simulink model "Mini_project_sim_2020"  (R2020b)
settings: Solver=ode113  StartTime=0.0  StopTime=10  FixedStep=0.001  RelTol=0.0001
values from neighbouring files (symbols this model uses):
  A = [0 1 0 0; 0.0290 0 7.0062 0; 0 0 0 1; -3.1991 0 0.1088 0]    [BallBeam3.m]
  B = [0; -4.332; 0; 47.7514]    [BallBeam3.m]
  C = [1 0 0 0;  0 0 1 0]    [BallBeam3.m]
  g = 9.81    [BallBeam3.m]
  ica = 0.1    [BallBeam3.m]
  icx = L/2    (= 0.21275)    [BallBeam3.m]
  J = 0.02    [BallBeam3.m]
  K = lqr(A,B,Q,R)    [BallBeam3.m]
  L = 0.4255    [BallBeam3.m]
  Lo = place(A', C', full_state_poles .* 10)'    [BallBeam3.m]
  m = 0.064    [BallBeam3.m]
  r = 0.0127    [BallBeam3.m]
  R = 1    [BallBeam3.m]
  step_input_value = 0.1    [BallBeam3.m]
undefined symbols (not defined in the file or in its folder): FSFB, K_Bar, Kd, Ki, Kp, observer_L, tau
libraries: simulink x2, dspsrcs4 x2
settings Model: Creator=jackg  LastModifiedBy=Andreas Wiedholz
settings SolverCC: MaxConsecutiveMinStep=500
settings DebuggingCC: SFMachineParentedDataDiag=error  UnderSpecifiedDimensionMsg=warning

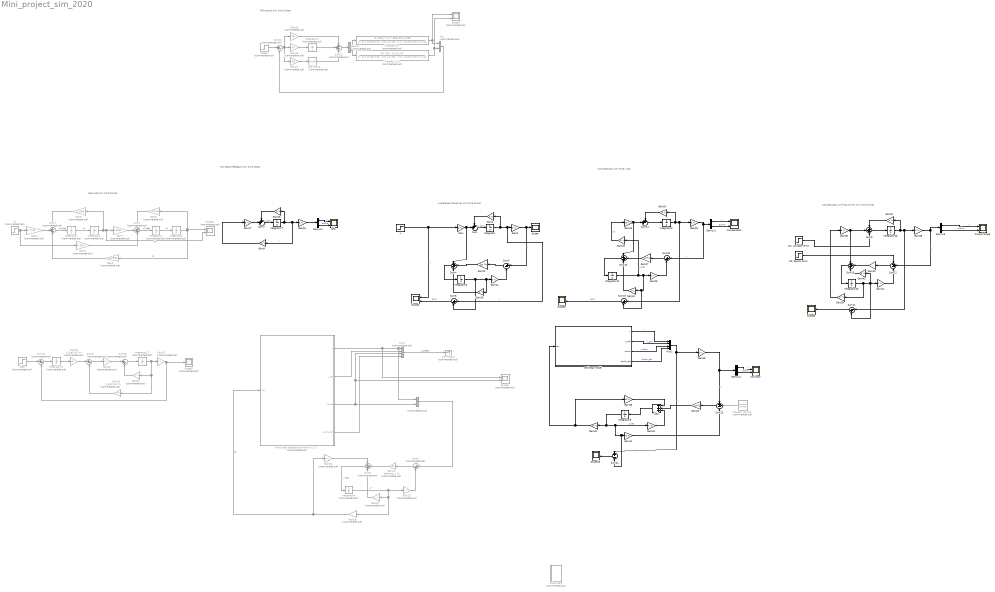
== system Mini_project_sim_2020 ==
  note: open loop sim time 10 sec
  note: Full State Feedback sim time 10sec
  note: Luenberger Observer sim time 10 sec
  note: Compensator sim time 1 sec
  note: Compensator with S/A errors sim time 10 sec
  note: PID control sim time 10sec
  AZ- Actuator error : Step  Time=0  After=[0; 0; 0.01; 0]  SampleTime=0
  Add : Sum  Inputs=+++
  Demux : Demux  Commented=on  Outputs=2
  Demux{1..4} (4 alike) : Demux  Outputs=2
  Derivative : Derivative  Commented=on
  Gain{,17,23,35..36} (5 alike) : Gain  Gain=B  Multiplication=Matrix(K*u)
  Gain{1,10,15,24,34,37,42..43} (8 alike) : Gain  Gain=A  Multiplication=Matrix(K*u)
  Gain{2,11,16,25,28,38,41,44,49} (9 alike) : Gain  Gain=C  Multiplication=Matrix(K*u)
  Gain{12,22,27,40} (4 alike) : Gain  Gain=Lo  Multiplication=Matrix(K*u)
  Gain13 : Gain  Commented=on  Gain=C  Multiplication=Matrix(K*u)
  Gain14 : Gain  Commented=on  Gain=observer_L  Multiplication=Matrix(K*u)
  Gain18 : Gain  Commented=on  Gain=B  Multiplication=Matrix(K*u)
  Gain19 : Gain  Commented=on  Gain=-FSFB  Multiplication=Matrix(K*u)
  Gain20 : Gain  Commented=on  Gain=A  Multiplication=Matrix(K*u)
  Gain{9,26,39,48} (4 alike) : Gain  Gain=-K  Multiplication=Matrix(K*u)
  Gain29 : Gain  Commented=on  Gain=K_Bar(5:6)  Multiplication=Matrix(K*u)
  Gain3 : Gain  Commented=on  Gain=3.1991
  Gain30 : Gain  Commented=on  Gain=B  Multiplication=Matrix(K*u)
  Gain31 : Gain  Commented=on  Gain=C  Multiplication=Matrix(K*u)
  Gain32 : Gain  Commented=on  Gain=A  Multiplication=Matrix(K*u)
  Gain33 : Gain  Commented=on  Gain=K_Bar(1:4)  Multiplication=Matrix(K*u)
  Gain4 : Gain  Commented=on  Gain=47.7514
  Gain45 : Gain  Commented=on  Gain=Kp
  Gain46 : Gain  Commented=on  Gain=Ki
  Gain47 : Gain  Commented=on  Gain=Kd
  Gain5 : Gain  Commented=on  Gain=0.1088
  Gain6 : Gain  Commented=on  Gain=4.332
  Gain7 : Gain  Commented=on  Gain=7.0062
  Gain8 : Gain  Commented=on  Gain=0.0290
  Integrator : Integrator
  Integrator{1..4,11..12,17} (7 alike) : Integrator  Commented=on
  Integrator10 : Integrator  InitialCondition=[0.1;0;0;0]
  Integrator15 : Integrator  InitialCondition=[0.1,0,0,0]
  Integrator16 : Integrator  InitialCondition=[icx;0;ica;0]
  Integrator5 : Integrator
  Integrator6 : Integrator  Commented=on  InitialCondition=[0;0;0;0]
  Integrator7 : Integrator  InitialCondition=[icx; 0;ica;0]
  Integrator8 : Integrator  InitialCondition=[0.1;0;0;0]
  Integrator9 : Integrator  InitialCondition=[icx;0;ica;0]
  Mux : Mux  Commented=on  Inputs=2
  Mux1 : Mux  Commented=on
  Mux2 : Mux
  "Non-Linear equations of motion 1 & 2 " : Subsystem  Commented=on
  Output Scope : Scope  NumInputPorts=2
  Random Source : dspsrcs4/Random Source  Commented=on  SrcType=Uniform  NormMethod=Ziggurat  CltLength=12  MinVal=[-0.01; -0.01]  MaxVal=[0.01; 0.01]  MeanVal=0  VarVal=1  RepMode=Not repeatable  rawSeed=1  IsInherit=off  SampMode=Discrete  SampTime=1  SampFrame=1  DataType=Double  OutComplex=Real  OutputFrames=off
  Scope{,6,8,10} (4 alike) : Scope
  Scope1 : Scope  Commented=on  NumInputPorts=2
  Scope2 : Scope  NumInputPorts=2
  Scope3 : Scope  Commented=on
  Scope5 : Scope  Commented=on  NumInputPorts=2
  Scope9 : Scope  Commented=on  NumInputPorts=4
  Step : Step  Commented=on  After=R  SampleTime=0
  Step3 : Step  Commented=on  SampleTime=0
  Subsystem : Subsystem  Commented=on
  Sum : Sum  Inputs=++|
  Sum1 : Sum  Commented=on  Inputs=++-
  Sum10 : Sum  Inputs=+++
  Sum11 : Sum  Inputs=|-+
  Sum12 : Sum  Inputs=-+-
  Sum13 : Sum  Inputs=++-
  Sum14 : Sum  Inputs=++|
  Sum15 : Sum  Inputs=+++
  Sum{3,16..17,21} (4 alike) : Sum  Commented=on  Inputs=|+-
  Sum18 : Sum  Commented=on  Inputs=|++
  Sum19 : Sum  Inputs=|+-
  Sum2 : Sum  Commented=on  Inputs=++-
  Sum20 : Sum  Inputs=|+-
  Sum22 : Sum  Commented=on  Inputs=+++
  Sum24 : Sum  Inputs=+-
  Sum4 : Sum  Inputs=+++
  Sum5 : Sum  Inputs=|+-  OutDataTypeStr=Inherit: Same as accumulator
  Sum6 : Sum  Inputs=|+-
  Sum7 : Sum  Inputs=++|
  Sum8 : Sum  Commented=on  Inputs=+++
  Sum9 : Sum  Inputs=++-
  Terminator : Terminator  Commented=on
  Transfer Fcn : TransferFcn  Commented=on  Numerator=[-4.332 7.69e-15 335]  Denominator=[1 -3.553e-15 -0.1378 1.332e-14 22.42]
  Transfer Fcn1 : TransferFcn  Commented=on  Numerator=[47.75 0 12.47]  Denominator=[1 -3.553e-15 -0.1378 1.332e-14 22.42]
  ZS- Sensor error : Step  Time=0  After=[-0.05 0]  SampleTime=0
  compensator : Scope  NumInputPorts=2
  fsfb : Scope  NumInputPorts=2
  nonlinear : Scope  NumInputPorts=2
  nonlinear model : Subsystem
  u : Step  After=step_input_value  SampleTime=0
  u1 : Step  Commented=on  SampleTime=0
  y : Mux  Commented=on  Inputs=2
  wires:
  Integrator/1 -> Sum6/1, Gain2/1, Gain1/1  "x"
  Sum/1 -> Integrator/1  "x_dot"
  Gain1/1 -> Sum/1
  Gain/1 -> Sum4/1, Sum/2
  Gain2/1 -> Sum5/1, Scope/1  "y"
  Integrator1/1 -> Integrator2/1  "x4"
  Integrator2/1 -> Scope1/2, Gain7/1, Gain5/1  "x3"
  Integrator3/1 -> Integrator4/1  "x2"
  Sum1/1 -> Integrator1/1  "x4_dot"
  Integrator4/1 -> Scope1/1, Gain8/1, Gain3/1  "x1"
  Gain3/1 -> Sum1/3
  Gain4/1 -> Sum1/2
  u1/1 -> Gain6/1, Gain4/1
  Gain5/1 -> Sum1/1
  Sum2/1 -> Integrator3/1  "x2_dot"
  Gain6/1 -> Sum2/3
  Gain7/1 -> Sum2/2
  Gain8/1 -> Sum2/1
  u/1 -> Gain/1, Scope2/1  "u"
  Integrator5/1 -> Sum6/2, Gain10/1, Gain11/1
  Gain11/1 -> Sum5/2
  Sum5/1 -> Gain12/1
  Sum4/1 -> Integrator5/1
  Sum6/1 -> Scope2/2  "error"
  Gain10/1 -> Sum4/3
  Gain12/1 -> Sum4/2
  Integrator7/1 -> Gain9/1, Gain16/1, Gain15/1  "x"
  Sum7/1 -> Integrator7/1  "x_dot"
  Gain15/1 -> Sum7/1
  Gain17/1 -> Sum7/2
  Step/1 -> Sum16/1
  Sum16/1 -> Integrator11/1
  Integrator11/1 -> Gain29/1
  Gain29/1 -> Sum17/1
  Sum17/1 -> Gain30/1
  Gain30/1 -> Sum18/1
  Sum18/1 -> Integrator12/1
  Integrator12/1 -> Gain33/1, Gain32/1, Gain31/1
  Gain32/1 -> Sum18/2
  Gain31/1 -> Scope3/1, Sum16/2
  Gain33/1 -> Sum17/2
  Gain23/1 -> Sum15/1, Sum14/2
  Gain24/1 -> Sum14/1
  Sum14/1 -> Integrator9/1
  Integrator9/1 -> Gain24/1, Sum19/1, Gain25/1
  Gain25/1 -> Demux1/1, Sum20/1  "y"
  Gain27/1 -> Sum15/2
  Sum20/1 -> Gain27/1
  Gain28/1 -> Sum20/2
  Integrator10/1 -> Gain34/1, Sum19/2, Gain28/1, Gain26/1  "x_hat"
  Sum15/1 -> Integrator10/1
  Gain34/1 -> Sum15/3
  Sum19/1 -> Scope8/1  "error"
  Sum11/1 -> Scope6/1
  Gain42/1 -> Sum10/3
  Sum10/1 -> Integrator15/1
  Integrator15/1 -> Sum11/2, Gain42/1, Gain41/1, Gain39/1
  Sum12/1 -> Gain40/1
  Gain40/1 -> Sum10/2
  Gain38/1 -> Sum12/2, Demux3/1  "y"
  Integrator16/1 -> Gain38/1, Sum11/1, Gain37/1
  Sum9/1 -> Integrator16/1
  Gain37/1 -> Sum9/1
  Gain36/1 -> Sum9/2, Sum10/1
  Gain39/1 -> Gain36/1
  AZ- Actuator error/1 -> Sum9/3
  Gain41/1 -> Sum12/3
  ZS- Sensor error/1 -> Sum12/1
  Demux/2 -> Transfer Fcn1/1
  Demux/1 -> Transfer Fcn/1
  Transfer Fcn/1 -> Scope5/1, Mux/1
  Transfer Fcn1/1 -> Scope5/2, Mux/2
  Mux/1 -> Sum21/2
  Step3/1 -> Sum21/1
  Sum22/1 -> Demux/1
  Sum21/1 -> Gain45/1, Gain47/1, Gain46/1
  Gain47/1 -> Derivative/1
  Derivative/1 -> Sum22/3
  Integrator17/1 -> Sum22/2
  Gain45/1 -> Sum22/1
  Gain46/1 -> Integrator17/1
  Demux1/2 -> compensator/2  "alpha"
  Gain16/1 -> Demux2/1  "y"
  Demux2/1 -> fsfb/1  "x"
  Demux2/2 -> fsfb/2  "alpha"
  Demux1/1 -> compensator/1  "x"
  Gain9/1 -> Gain17/1
  Gain26/1 -> Gain23/1  "Lin"
  Demux3/1 -> Output Scope/1  "x"
  Demux3/2 -> Output Scope/2  "alpha"
  "Non-Linear equations of motion 1 & 2 "/1(x) -> Scope9/2, y/1, Mux1/1
  "Non-Linear equations of motion 1 & 2 "/2(x_dot) -> Mux1/2
  "Non-Linear equations of motion 1 & 2 "/3(alpha) -> y/2, Mux1/3, Scope9/3
  "Non-Linear equations of motion 1 & 2 "/4(alpha_dot) -> Mux1/4
  Mux1/1 -> Terminator/1  "x_vector"
  Gain13/1 -> Sum3/2
  Sum3/1 -> Gain14/1
  y/1 -> Sum3/1
  Gain14/1 -> Sum8/2
  Gain18/1 -> Sum8/1
  Gain19/1 -> Gain18/1, "Non-Linear equations of motion 1 & 2 "/1(Tau)  "NL"
  Integrator6/1 -> Gain13/1, Gain20/1, Gain19/1  "x^"
  Sum8/1 -> Integrator6/1  "x^dot"
  Gain20/1 -> Sum8/3
  Gain48/1 -> Gain35/1, nonlinear model/1(tau)
  Sum13/1 -> Gain22/1
  Integrator8/1 -> Gain43/1, Sum24/2, Gain44/1, Gain48/1  "x_hat"
  Gain44/1 -> Sum13/3
  nonlinear model/3(alpha) -> Mux2/3  "alpha"
  nonlinear model/4(alpha_dot) -> Mux2/4  "alpha_dot"
  Sum24/1 -> Scope10/1
  nonlinear model/2(x_dot) -> Mux2/2  "x_dot"
  nonlinear model/1(x) -> Mux2/1  "x"
  Mux2/1 -> Gain49/1, Sum24/1  "x"
  Gain35/1 -> Add/1
  Gain22/1 -> Add/2
  Gain43/1 -> Add/3
  Add/1 -> Integrator8/1
  Gain49/1 -> Sum13/1, Demux4/1  "y"
  Demux4/1 -> nonlinear/1  "x"
  Demux4/2 -> nonlinear/2  "alpha"
  Random Source/1 -> Sum13/2

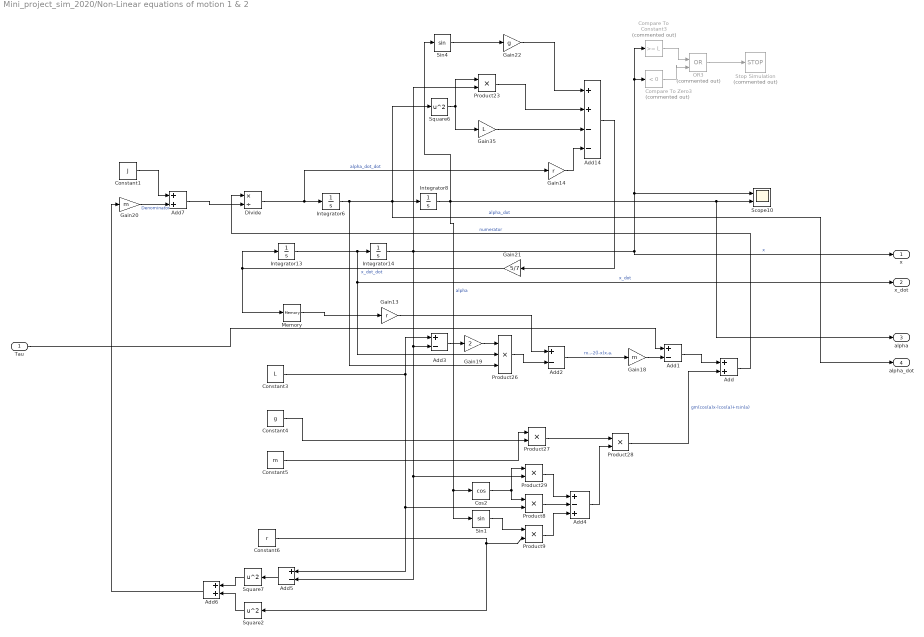
== system Mini_project_sim_2020/Non-Linear equations of motion 1 & 2  ==
  Tau : Inport
  Add : Sum
  Add{1..3,5} (4 alike) : Sum  Inputs=+-
  Add14 : Sum  Inputs=++--
  Add4 : Sum  Inputs=+-+
  Add6 : Sum
  Add7 : Sum
  Compare To Constant3 : simulink/Logic and Bit Operations/Compare To Constant  Commented=on  relop=>=  const=L  OutDataTypeStr=boolean
  Compare To Zero3 : simulink/Logic and Bit Operations/Compare To Zero  Commented=on  relop=<  OutDataTypeStr=boolean
  Constant1 : Constant  Value=J
  Constant3 : Constant  Value=L
  Constant4 : Constant  Value=g
  Constant5 : Constant  Value=m
  Constant6 : Constant  Value=r
  Cos2 : Trigonometry  Operator=cos
  Divide : Product  Inputs=*/
  Gain13 : Gain  Gain=r
  Gain14 : Gain  Gain=r
  Gain18 : Gain  Gain=m
  Gain19 : Gain  Gain=2
  Gain20 : Gain  Gain=m
  Gain21 : Gain  Gain=5/7
  Gain22 : Gain  Gain=g
  Gain35 : Gain  Gain=L
  Integrator13 : Integrator
  Integrator14 : Integrator  InitialCondition=L/2
  Integrator6 : Integrator
  Integrator8 : Integrator  InitialCondition=0.1
  Memory : Memory
  OR3 : Logic  Commented=on  Operator=OR  IconShape=distinctive  AllPortsSameDT=off  OutDataTypeStr=boolean
  Product{8..9,23,27..29} (6 alike) : Product
  Product26 : Product  Inputs=3
  Scope10 : Scope  NumInputPorts=2
  Sin1 : Trigonometry
  Sin4 : Trigonometry
  Square2 : Math  Operator=square  SaturateOnIntegerOverflow=on
  Square6 : Math  Operator=square  SaturateOnIntegerOverflow=on
  Square7 : Math  Operator=square  SaturateOnIntegerOverflow=on
  Stop Simulation : Stop  Commented=on
  x : Outport
  x_dot : Outport  Port=2
  alpha : Outport  Port=3
  alpha_dot : Outport  Port=4
  wires:
  Square7/1 -> Add6/1
  Integrator6/1 -> Product26/3, alpha_dot/1, Square6/1, Integrator8/1  "alpha_dot"
  Add7/1 -> Divide/2
  Divide/1 -> Gain14/1, Integrator6/1  "alpha_dot_dot"
  Sin4/1 -> Gain22/1
  Integrator8/1 -> Sin1/1, Cos2/1, alpha/1, Scope10/2, Sin4/1  "alpha"
  Add/1 -> Divide/1  "numerator"
  Gain35/1 -> Add14/3
  Gain14/1 -> Add14/4
  Compare To Constant3/1 -> OR3/1
  Square2/1 -> Add6/2
  Integrator14/1 -> Compare To Zero3/1, Compare To Constant3/1, Scope10/1, x/1, Product23/2, Add5/2, Product29/2, Add3/2  "x"
  Constant4/1 -> Product27/2
  OR3/1 -> Stop Simulation/1
  Constant6/1 -> Square2/1, Product9/2
  Gain19/1 -> Product26/1
  Integrator13/1 -> Integrator14/1, x_dot/1, Product26/2  "x_dot"
  Gain13/1 -> Add2/1
  Add1/1 -> Add/1
  Product9/1 -> Add4/3
  Constant5/1 -> Product27/1
  Gain20/1 -> Add7/2  "Denominator"
  Gain21/1 -> Memory/1, Integrator13/1  "x_dot_dot"
  Constant1/1 -> Add7/1
  Constant3/1 -> Add3/1, Add5/1, Product8/2
  Add5/1 -> Square7/1
  Product29/1 -> Add4/1
  Add6/1 -> Gain20/1
  Cos2/1 -> Product29/1, Product8/1
  Gain18/1 -> Add1/2
  Compare To Zero3/1 -> OR3/2
  Product8/1 -> Add4/2
  Add14/1 -> Gain21/1
  Add4/1 -> Product28/2
  Square6/1 -> Gain35/1, Product23/1
  Product26/1 -> Add2/2
  Sin1/1 -> Product9/1
  Add3/1 -> Gain19/1
  Product23/1 -> Add14/2
  Product27/1 -> Product28/1
  Gain22/1 -> Add14/1
  Add2/1 -> Gain18/1  "rx..-2(l-x)x.a."
  Product28/1 -> Add/2  "gm(cos(a)x-lcos(a)+rsin(a)"
  Memory/1 -> Gain13/1
  Tau/1 -> Add1/1

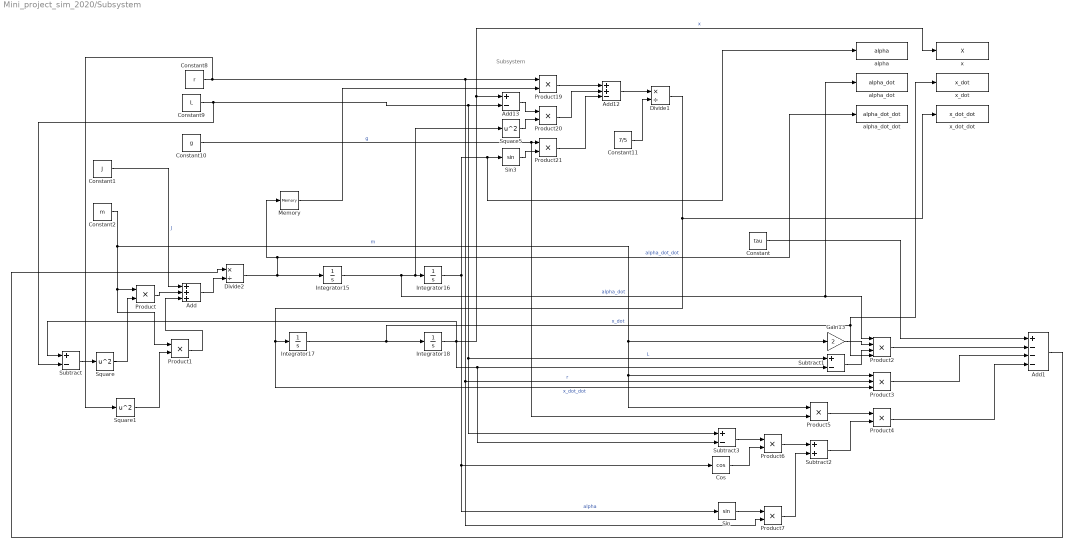
== system Mini_project_sim_2020/Subsystem ==
  note: Subsystem
  Add : Sum  Inputs=+++
  Add1 : Sum  Inputs=+---
  Add12 : Sum  Inputs=++-
  Add13 : Sum  Inputs=+-
  Constant : Constant  Value=tau
  Constant1 : Constant  Value=J
  Constant10 : Constant  Value=g
  Constant11 : Constant  Value=7/5
  Constant2 : Constant  Value=m
  Constant8 : Constant  Value=r
  Constant9 : Constant  Value=L
  Cos : Trigonometry  Operator=cos
  Divide1 : Product  Inputs=*/
  Divide2 : Product  Inputs=*/
  Gain13 : Gain  Gain=2
  Integrator{15..18} (4 alike) : Integrator
  Memory : Memory
  Product{,1,4..7,19..21} (9 alike) : Product
  Product2 : Product  Inputs=4
  Product3 : Product  Inputs=3
  Sin : Trigonometry
  Sin3 : Trigonometry
  Square : Math  Operator=square  SaturateOnIntegerOverflow=on
  Square1 : Math  Operator=square  SaturateOnIntegerOverflow=on
  Square5 : Math  Operator=square  SaturateOnIntegerOverflow=on
  Subtract : Sum  Inputs=+-
  Subtract1 : Sum  Inputs=+-
  Subtract2 : Sum
  Subtract3 : Sum  Inputs=+-
  alpha : ToWorkspace  VariableName=alpha  SaveFormat=Timeseries  SampleTime=-1
  alpha_dot : ToWorkspace  VariableName=alpha_dot  SaveFormat=Timeseries  SampleTime=-1
  alpha_dot_dot : ToWorkspace  VariableName=alpha_dot_dot  SaveFormat=Timeseries  SampleTime=-1
  x : ToWorkspace  VariableName=X  SaveFormat=Timeseries  SampleTime=-1
  x_dot : ToWorkspace  VariableName=x_dot  SaveFormat=Timeseries  SampleTime=-1
  x_dot_dot : ToWorkspace  VariableName=x_dot_dot  SaveFormat=Timeseries  SampleTime=-1
  wires:
  Integrator15/1 -> alpha_dot/1, Product2/1, Square5/1, Integrator16/1  "alpha_dot"
  Divide2/1 -> Memory/1, alpha_dot_dot/1, Integrator15/1  "alpha_dot_dot"
  Constant8/1 -> Square1/1, Product7/2, Product3/2, Product19/1  "r"
  Subtract/1 -> Square/1
  Sin3/1 -> Product21/2
  Integrator18/1 -> Subtract3/2, Subtract1/2, Subtract/1, x/1, Add13/1  "x"
  Product2/1 -> Add1/2
  Constant1/1 -> Add/1  "J"
  Divide1/1 -> x_dot_dot/1, Product3/3, Integrator17/1  "x_dot_dot"
  Square1/1 -> Product1/2
  Add13/1 -> Product20/1
  Constant10/1 -> Product5/2, Product21/1  "g"
  Constant9/1 -> Subtract/2, Subtract3/1, Subtract1/1, Add13/2  "L"
  Constant/1 -> Add1/1
  Square/1 -> Product/2
  Gain13/1 -> Product2/2
  Product7/1 -> Subtract2/2
  Constant2/1 -> Product5/1, Product3/1, Gain13/1, Product1/1, Product/1  "m"
  Constant11/1 -> Divide1/2
  Product3/1 -> Add1/3
  Product/1 -> Add/2
  Integrator16/1 -> alpha/1, Sin3/1, Cos/1, Sin/1  "alpha"
  Integrator17/1 -> x_dot/1, Product2/4, Integrator18/1  "x_dot"
  Subtract3/1 -> Product6/1
  Product21/1 -> Add12/3
  Cos/1 -> Product6/2
  Product19/1 -> Add12/1
  Product6/1 -> Subtract2/1
  Sin/1 -> Product7/1
  Product1/1 -> Add/3
  Subtract2/1 -> Product4/2
  Add12/1 -> Divide1/1
  Product20/1 -> Add12/2
  Add/1 -> Divide2/2
  Product4/1 -> Add1/4
  Square5/1 -> Product20/2
  Product5/1 -> Product4/1
  Add1/1 -> Divide2/1
  Subtract1/1 -> Product2/3
  Memory/1 -> Product19/2

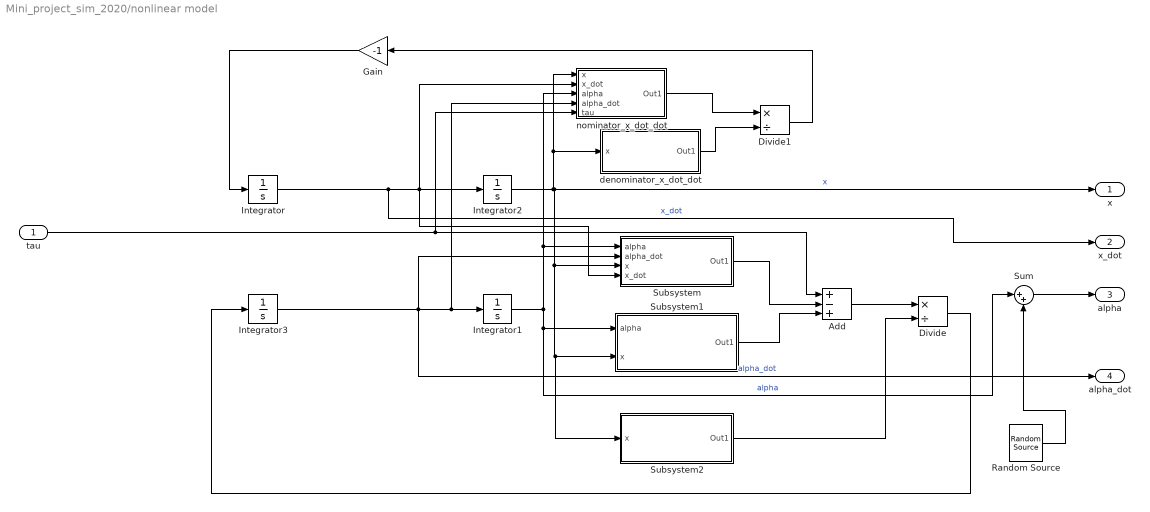
== system Mini_project_sim_2020/nonlinear model ==
  tau : Inport
  Add : Sum  Inputs=+-+
  Divide : Product  Inputs=*/
  Divide1 : Product  Inputs=*/
  Gain : Gain  Gain=-1
  Integrator : Integrator
  Integrator1 : Integrator  InitialCondition=0.1
  Integrator2 : Integrator  InitialCondition=L/2
  Integrator3 : Integrator
  Random Source : dspsrcs4/Random Source  SrcType=Uniform  NormMethod=Ziggurat  CltLength=12  MinVal=-0.01  MaxVal=0.02  MeanVal=0  VarVal=1  RepMode=Not repeatable  rawSeed=1  IsInherit=off  SampMode=Discrete  SampTime=1  SampFrame=1  DataType=Double  OutComplex=Real  OutputFrames=off
  Subsystem : Subsystem
      mask Display: disp('m(r(5gsin(alpha)...))')
  Subsystem1 : Subsystem
      mask Display: disp('gm(cos(alpha)...)')
  Subsystem2 : Subsystem
      mask Display: disp('denominator')
  Sum : Sum  Inputs=|++
  denominator_x_dot_dot : Subsystem
      mask Display: disp('denominator')
  nominator_x_dot_dot : Subsystem
      mask Display: disp('nominator')
  x : Outport
  x_dot : Outport  Port=2
  alpha : Outport  Port=3
  alpha_dot : Outport  Port=4
  wires:
  Integrator/1 -> x_dot/1, nominator_x_dot_dot/2(x_dot), Subsystem/4(x_dot), Integrator2/1  "x_dot"
  Integrator3/1 -> alpha_dot/1, nominator_x_dot_dot/4(alpha_dot), Integrator1/1, Subsystem/2(alpha_dot)  "alpha_dot"
  Integrator1/1 -> Sum/1, Subsystem1/1(alpha), nominator_x_dot_dot/3(alpha), Subsystem/1(alpha)  "alpha"
  Integrator2/1 -> x/1, Subsystem/3(x), Subsystem2/1(x), Subsystem1/2(x), denominator_x_dot_dot/1(x), nominator_x_dot_dot/1(x)  "x"
  tau/1 -> nominator_x_dot_dot/5(tau), Add/1
  Subsystem/1(Out1) -> Add/2
  Subsystem1/1(Out1) -> Add/3
  Add/1 -> Divide/1
  Subsystem2/1(Out1) -> Divide/2
  Divide/1 -> Integrator3/1
  nominator_x_dot_dot/1(Out1) -> Divide1/1
  denominator_x_dot_dot/1(Out1) -> Divide1/2
  Divide1/1 -> Gain/1
  Gain/1 -> Integrator/1
  Sum/1 -> alpha/1
  Random Source/1 -> Sum/2

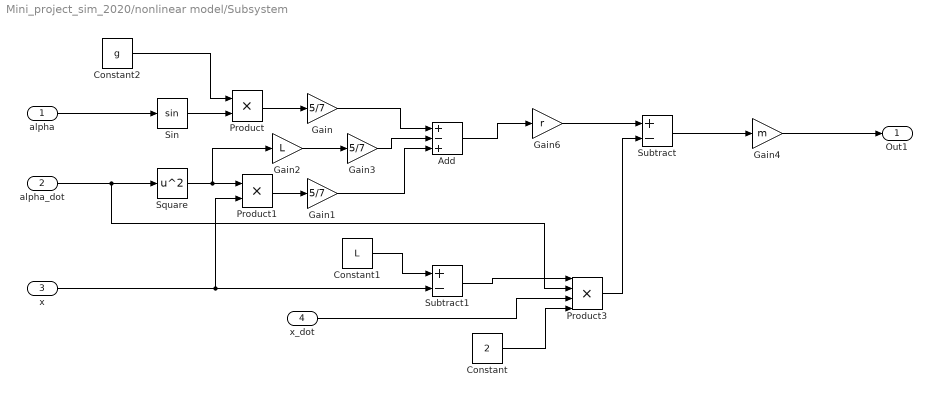
== system Mini_project_sim_2020/nonlinear model/Subsystem ==
  alpha : Inport
  alpha_dot : Inport  Port=2
  x : Inport  Port=3
  x_dot : Inport  Port=4
  Add : Sum  Inputs=+-+
  Constant : Constant  Value=2
  Constant1 : Constant  Value=L
  Constant2 : Constant  Value=g
  Gain : Gain  Gain=5/7
  Gain1 : Gain  Gain=5/7
  Gain2 : Gain  Gain=L
  Gain3 : Gain  Gain=5/7
  Gain4 : Gain  Gain=m
  Gain6 : Gain  Gain=r
  Product : Product
  Product1 : Product
  Product3 : Product  Inputs=4
  Sin : Trigonometry
  Square : Math  Operator=square  SaturateOnIntegerOverflow=on
  Subtract : Sum  Inputs=+-
  Subtract1 : Sum  Inputs=+-
  Out1 : Outport
  wires:
  alpha_dot/1 -> Product3/2, Square/1
  alpha/1 -> Sin/1
  Sin/1 -> Product/2
  Constant2/1 -> Product/1
  Product/1 -> Gain/1
  Square/1 -> Gain2/1, Product1/1
  x/1 -> Product1/2, Subtract1/2
  Product1/1 -> Gain1/1
  Gain2/1 -> Gain3/1
  Gain/1 -> Add/1
  Gain3/1 -> Add/2
  Gain1/1 -> Add/3
  Gain4/1 -> Out1/1
  Gain6/1 -> Subtract/1
  Constant1/1 -> Subtract1/1
  Subtract1/1 -> Product3/1
  x_dot/1 -> Product3/3
  Product3/1 -> Subtract/2
  Subtract/1 -> Gain4/1
  Add/1 -> Gain6/1
  Constant/1 -> Product3/4

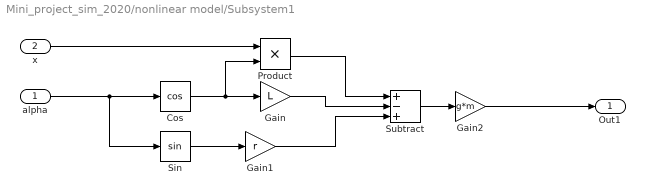
== system Mini_project_sim_2020/nonlinear model/Subsystem1 ==
  alpha : Inport
  x : Inport  Port=2
  Cos : Trigonometry  Operator=cos
  Gain : Gain  Gain=L
  Gain1 : Gain  Gain=r
  Gain2 : Gain  Gain=g*m
  Product : Product
  Sin : Trigonometry
  Subtract : Sum  Inputs=+-+
  Out1 : Outport
  wires:
  alpha/1 -> Sin/1, Cos/1
  x/1 -> Product/1
  Cos/1 -> Gain/1, Product/2
  Product/1 -> Subtract/1
  Gain/1 -> Subtract/2
  Sin/1 -> Gain1/1
  Gain1/1 -> Subtract/3
  Subtract/1 -> Gain2/1
  Gain2/1 -> Out1/1

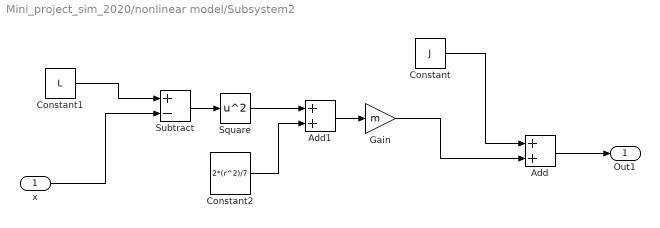
== system Mini_project_sim_2020/nonlinear model/Subsystem2 ==
  x : Inport
  Add : Sum
  Add1 : Sum
  Constant : Constant  Value=J
  Constant1 : Constant  Value=L
  Constant2 : Constant  Value=2*(r^2)/7
  Gain : Gain  Gain=m
  Square : Math  Operator=square  SaturateOnIntegerOverflow=on
  Subtract : Sum  Inputs=+-
  Out1 : Outport
  wires:
  Add/1 -> Out1/1
  Constant/1 -> Add/1
  Constant1/1 -> Subtract/1
  x/1 -> Subtract/2
  Subtract/1 -> Square/1
  Square/1 -> Add1/1
  Constant2/1 -> Add1/2
  Add1/1 -> Gain/1
  Gain/1 -> Add/2

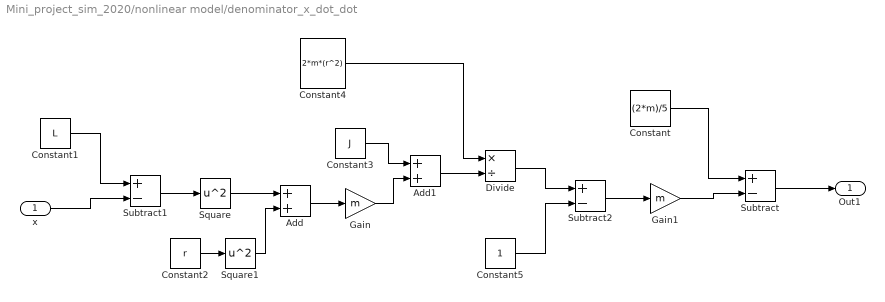
== system Mini_project_sim_2020/nonlinear model/denominator_x_dot_dot ==
  x : Inport
  Add : Sum
  Add1 : Sum
  Constant : Constant  Value=(2*m)/5
  Constant1 : Constant  Value=L
  Constant2 : Constant  Value=r
  Constant3 : Constant  Value=J
  Constant4 : Constant  Value=2*m*(r^2)
  Constant5 : Constant
  Divide : Product  Inputs=*/
  Gain : Gain  Gain=m
  Gain1 : Gain  Gain=m
  Square : Math  Operator=square  SaturateOnIntegerOverflow=on
  Square1 : Math  Operator=square  SaturateOnIntegerOverflow=on
  Subtract : Sum  Inputs=+-
  Subtract1 : Sum  Inputs=+-
  Subtract2 : Sum  Inputs=+-
  Out1 : Outport
  wires:
  Subtract/1 -> Out1/1
  Constant/1 -> Subtract/1
  x/1 -> Subtract1/2
  Constant1/1 -> Subtract1/1
  Subtract1/1 -> Square/1
  Square/1 -> Add/1
  Constant2/1 -> Square1/1
  Square1/1 -> Add/2
  Add/1 -> Gain/1
  Gain/1 -> Add1/2
  Constant3/1 -> Add1/1
  Add1/1 -> Divide/2
  Constant4/1 -> Divide/1
  Constant5/1 -> Subtract2/2
  Divide/1 -> Subtract2/1
  Subtract2/1 -> Gain1/1
  Gain1/1 -> Subtract/2

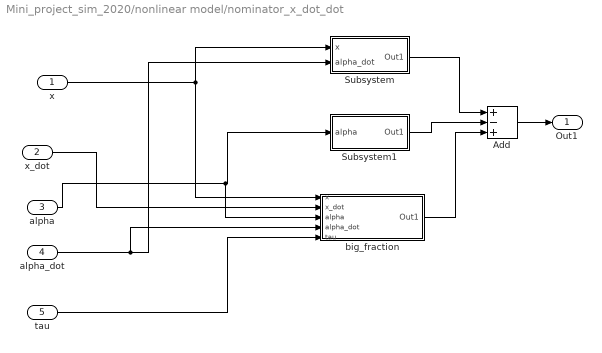
== system Mini_project_sim_2020/nonlinear model/nominator_x_dot_dot ==
  x : Inport
  x_dot : Inport  Port=2
  alpha : Inport  Port=3
  alpha_dot : Inport  Port=4
  tau : Inport  Port=5
  Add : Sum  Inputs=+-+
  Subsystem : Subsystem
      mask Display: disp('m(l-x)(a_dot)^2')
  Subsystem1 : Subsystem
      mask Display: disp('gmsin(alpha)')
  big_fraction : Subsystem
      mask Display: disp('fraction')
  Out1 : Outport
  wires:
  big_fraction/1(Out1) -> Add/3
  Subsystem1/1(Out1) -> Add/2
  Subsystem/1(Out1) -> Add/1
  x/1 -> big_fraction/1(x), Subsystem/1(x)
  alpha_dot/1 -> big_fraction/4(alpha_dot), Subsystem/2(alpha_dot)
  alpha/1 -> big_fraction/3(alpha), Subsystem1/1(alpha)
  x_dot/1 -> big_fraction/2(x_dot)
  tau/1 -> big_fraction/5(tau)
  Add/1 -> Out1/1

== system Mini_project_sim_2020/nonlinear model/nominator_x_dot_dot/Subsystem ==
  x : Inport
  alpha_dot : Inport  Port=2
  Constant : Constant  Value=L
  Gain : Gain  Gain=m
  Product : Product
  Square : Math  Operator=square  SaturateOnIntegerOverflow=on
  Subtract : Sum  Inputs=+-
  Out1 : Outport
  wires:
  alpha_dot/1 -> Square/1
  x/1 -> Subtract/2
  Constant/1 -> Subtract/1
  Square/1 -> Product/2
  Subtract/1 -> Product/1
  Product/1 -> Gain/1
  Gain/1 -> Out1/1

== system Mini_project_sim_2020/nonlinear model/nominator_x_dot_dot/Subsystem1 ==
  alpha : Inport
  Gain : Gain  Gain=g
  Gain1 : Gain  Gain=m
  Sin : Trigonometry
  Out1 : Outport
  wires:
  alpha/1 -> Sin/1
  Sin/1 -> Gain/1
  Gain/1 -> Gain1/1
  Gain1/1 -> Out1/1

== system Mini_project_sim_2020/nonlinear model/nominator_x_dot_dot/big_fraction ==
  x : Inport
  x_dot : Inport  Port=2
  alpha : Inport  Port=3
  alpha_dot : Inport  Port=4
  tau : Inport  Port=5
  Divide : Product  Inputs=*/
  denominator : Subsystem
      mask Display: disp('denominator')
  nominator : Subsystem
      mask Display: disp('nominator')
  Out1 : Outport
  wires:
  denominator/1(Out1) -> Divide/2
  nominator/1(Out1) -> Divide/1
  Divide/1 -> Out1/1
  x/1 -> denominator/1(x), nominator/1(x)
  x_dot/1 -> nominator/2(x_dot)
  alpha/1 -> nominator/3(alpha)
  alpha_dot/1 -> nominator/4(alpha_dot)
  tau/1 -> nominator/5(tau)

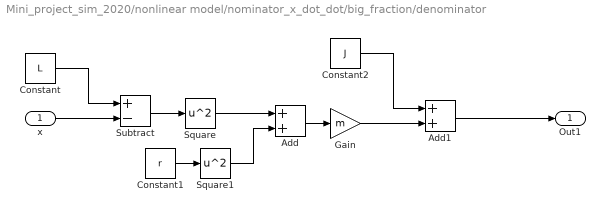
== system Mini_project_sim_2020/nonlinear model/nominator_x_dot_dot/big_fraction/denominator ==
  x : Inport
  Add : Sum
  Add1 : Sum
  Constant : Constant  Value=L
  Constant1 : Constant  Value=r
  Constant2 : Constant  Value=J
  Gain : Gain  Gain=m
  Square : Math  Operator=square  SaturateOnIntegerOverflow=on
  Square1 : Math  Operator=square  SaturateOnIntegerOverflow=on
  Subtract : Sum  Inputs=+-
  Out1 : Outport
  wires:
  x/1 -> Subtract/2
  Constant/1 -> Subtract/1
  Subtract/1 -> Square/1
  Square/1 -> Add/1
  Constant1/1 -> Square1/1
  Square1/1 -> Add/2
  Add/1 -> Gain/1
  Gain/1 -> Add1/2
  Constant2/1 -> Add1/1
  Add1/1 -> Out1/1

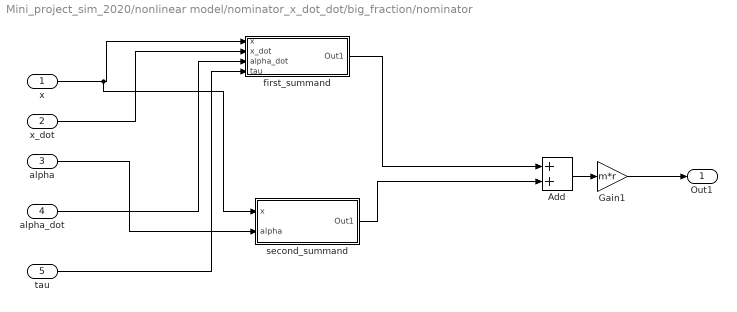
== system Mini_project_sim_2020/nonlinear model/nominator_x_dot_dot/big_fraction/nominator ==
  x : Inport
  x_dot : Inport  Port=2
  alpha : Inport  Port=3
  alpha_dot : Inport  Port=4
  tau : Inport  Port=5
  Add : Sum
  Gain1 : Gain  Gain=m*r
  first_summand : Subsystem
      mask Display: disp('first_summand')
  second_summand : Subsystem
      mask Display: disp('second_summand')
  Out1 : Outport
  wires:
  second_summand/1(Out1) -> Add/2
  first_summand/1(Out1) -> Add/1
  Add/1 -> Gain1/1
  x/1 -> second_summand/1(x), first_summand/1(x)
  x_dot/1 -> first_summand/2(x_dot)
  alpha_dot/1 -> first_summand/3(alpha_dot)
  alpha/1 -> second_summand/2(alpha)
  tau/1 -> first_summand/4(tau)
  Gain1/1 -> Out1/1

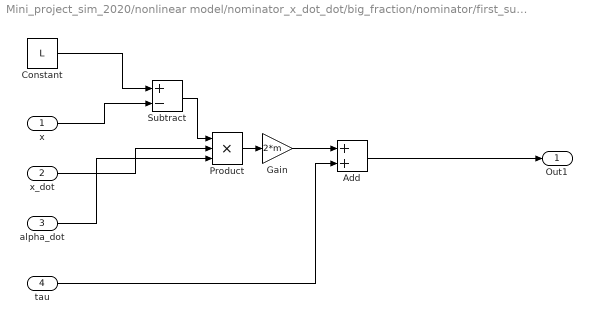
== system Mini_project_sim_2020/nonlinear model/nominator_x_dot_dot/big_fraction/nominator/first_summand ==
  x : Inport
  x_dot : Inport  Port=2
  alpha_dot : Inport  Port=3
  tau : Inport  Port=4
  Add : Sum
  Constant : Constant  Value=L
  Gain : Gain  Gain=2*m
  Product : Product  Inputs=3
  Subtract : Sum  Inputs=+-
  Out1 : Outport
  wires:
  Constant/1 -> Subtract/1
  x/1 -> Subtract/2
  Subtract/1 -> Product/1
  x_dot/1 -> Product/2
  alpha_dot/1 -> Product/3
  Product/1 -> Gain/1
  Gain/1 -> Add/1
  tau/1 -> Add/2
  Add/1 -> Out1/1

== system Mini_project_sim_2020/nonlinear model/nominator_x_dot_dot/big_fraction/nominator/second_summand ==
  x : Inport
  alpha : Inport  Port=2
  Add : Sum  Inputs=+-+
  Cos : Trigonometry  Operator=cos
  Gain : Gain  Gain=g*m
  Gain1 : Gain  Gain=r
  Gain2 : Gain  Gain=L
  Product : Product
  Sin : Trigonometry
  Out1 : Outport
  wires:
  Gain/1 -> Out1/1
  alpha/1 -> Sin/1, Cos/1
  Sin/1 -> Gain1/1
  Cos/1 -> Product/2, Gain2/1
  x/1 -> Product/1
  Product/1 -> Add/1
  Gain2/1 -> Add/2
  Gain1/1 -> Add/3
  Add/1 -> Gain/1
